simulink model "block1_simulink"  (R2025a)
settings: Solver=ode23tb  StartTime=0.0  StopTime=4  RelTol=1e-3
values from neighbouring files (symbols this model uses):
  C = 1.05 * C_min    (= -2.49234641954e-06)    [block1.m]
  G = 1.25/Vc_nom^2    (= 0.00882706023586)    [block1.m]
  I0_nom = P_nom/Vc_nom    (= 8.40336134454)    [block1.m]
  Il_nom = P_nom/(n*V0)    (= 8.77192982456)    [block1.m]
  KI = 0.5    [block1.m]
  KI_c = 200    [block1.m]
  Kp = 0.5    [block1.m]
  Kp_c = 500    [block1.m]
  L = 1.05 * L_min    (= -2.52e-06)    [block1.m]
  R = 3.75/Il_nom^2    (= 0.048735)    [block1.m]
  V0 = 12    [block1.m]
  Vc_nom = 11.9    [block1.m]
libraries: SignalEditorBlockLib x1
settings Model: Creator=arntzen  LastModifiedBy=Markus

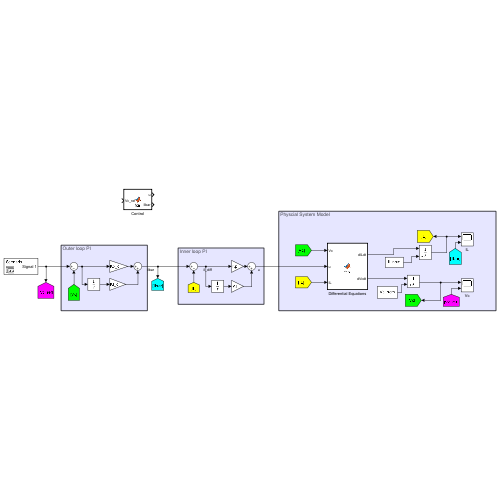
[thumbnail: Simulink's stored preview of the top-level diagram]
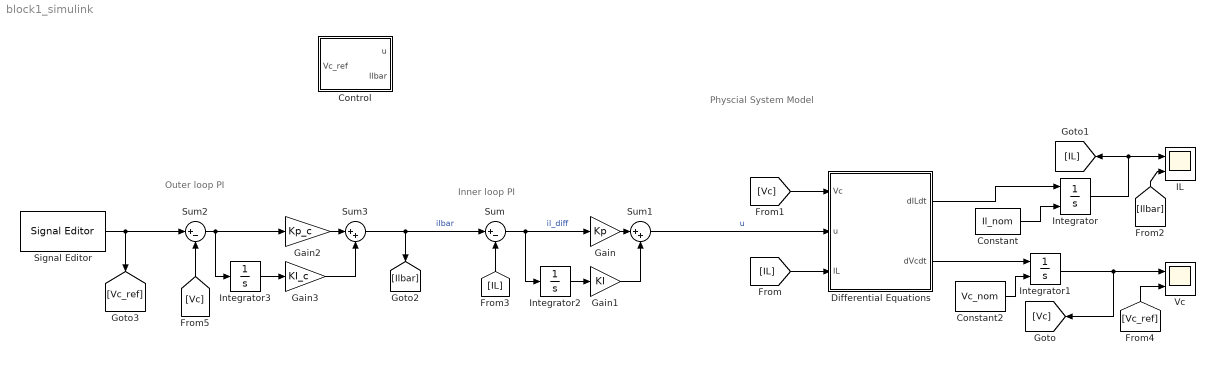
== system block1_simulink ==
  note: Inner loop PI
  note: Outer loop PI
  note: Physcial System Model
  Constant : Constant  Value=Il_nom
  Constant2 : Constant  Value=Vc_nom
  Control : MATLAB Function  TreatAsAtomicUnit=on
  Differential Equations : MATLAB Function  TreatAsAtomicUnit=on
  Gain : Gain  Gain=Kp
  Gain1 : Gain  Gain=KI
  Gain2 : Gain  Gain=Kp_c
  Gain3 : Gain  Gain=KI_c
  IL : Scope  NumInputPorts=2
      settings: ActiveDisplayYMinimum=-1164.660014247951  ActiveDisplayYMaximum=679.02179231657351
  Integrator : Integrator  InitialConditionSource=external
  Integrator1 : Integrator  InitialConditionSource=external
  Integrator2 : Integrator
  Integrator3 : Integrator
  Signal Editor : SignalEditorBlockLib/Signal Editor  FileName=DC_DC_Converter_SignalEditor.mat  ActiveScenario=Scenario  ActiveSignal=Signal 1  IsBus=off  OutputBusObjectStr=Bus: BusObject  SampleTime=0  Interpolate=off  ZeroCross=off  OutputAfterFinalValue=Setting to zero  Unit=inherit  PreserveSignalName=on  ApplySigPropsToAllScenarios=on  ApplySigPropsToAllSignals=off  SignalPropertySource=Dialog parameters
  Sum : Sum  Inputs=|+-
  Sum1 : Sum  Inputs=|++
  Sum2 : Sum  Inputs=|+-
  Sum3 : Sum  Inputs=|++
  Vc : Scope  NumInputPorts=2
      settings: ActiveDisplayYMinimum=9.7373470568963754  ActiveDisplayYMaximum=12.253765159244592
  wires:
  Differential Equations/1(dILdt) -> Integrator/1
  [IL] -> Differential Equations/3(IL)
  [Vc] -> Differential Equations/1(Vc)
  Constant/1 -> Integrator/2
  Integrator/1 -> [IL], IL/1
  Differential Equations/2(dVcdt) -> Integrator1/1
  Integrator1/1 -> [Vc], Vc/1
  Constant2/1 -> Integrator1/2
  [Vc_ref] -> Vc/2
  [Ilbar] -> IL/2
  Sum/1 -> Integrator2/1, Gain/1  "il_diff"
  [IL] -> Sum/2
  Gain/1 -> Sum1/1
  Gain1/1 -> Sum1/2
  Sum2/1 -> Gain2/1, Integrator3/1
  Signal Editor/1 -> Sum2/1, [Vc_ref]
  [Vc] -> Sum2/2
  Sum1/1 -> Differential Equations/2(u)  "u"
  Integrator3/1 -> Gain3/1
  Gain3/1 -> Sum3/2
  Gain2/1 -> Sum3/1
  Sum3/1 -> [Ilbar], Sum/1  "ilbar"
  Integrator2/1 -> Gain1/1

== matlab function block1_simulink/Control ==
  data: u output; V0 parameter; R parameter; G parameter; I0_nom parameter; Vc_ref input; Ilbar output
function [u, Ilbar] = fcn(V0, R, G, I0_nom, Vc_ref)

Ilbar = (V0 - sqrt(V0^2 - 4*R*(G*Vc_ref^2 + I0_nom*Vc_ref))) / (2*R);
u = 1 - (G*Vc_ref + I0_nom) / Ilbar;

== matlab function block1_simulink/Differential Equations ==
  data: R parameter; G parameter; V0 parameter; dILdt output; I0_nom parameter; dVcdt output; Vc input; u input; IL input; L parameter; C parameter
%function [dILdt, dVcdt] = fcn(R, C, L, V0, G, I0_nom, Vc_nom)
function [dILdt, dVcdt] = fcn(R,G,V0,I0_nom, Vc, u, IL, L, C)

dILdt = -R/L*IL - (1-u)/L*Vc + V0/L
dVcdt = -G/C*Vc + (1-u)/C*IL - I0_nom/C
